simulink model "gauss_mf1_2"  (Simulink 7.2)
settings: Solver=ode45  StartTime=0.0  StopTime=10.0  RelTol=1e-3
values from neighbouring files (symbols this model uses):
  fi_1_mu = -0.7664    [fuzzy_controller_5_gauss_params.m]
  fi_1_sigma = 0.1502    [fuzzy_controller_5_gauss_params.m]
settings Model: Creator=Student  LastModifiedBy=Student  CovModelRefEnable=off
settings DataIOCC: LimitDataPoints=off  SaveFormat=StructureWithTime
settings OptimizationCC: ExpressionDepthLimit=128
settings DebuggingCC: UnderspecifiedInitializationDetection=Simplified  MergeDetectMultiDrivingBlocksExec=error  SolverPrmCheckMsg=none  FcnCallInpInsideContextMsg=Enable All  StateNameClashWarn=none  StrictBusMsg=ErrorLevel1
settings HardwareCC: ProdIntDivRoundTo=Zero  ProdEndianess=LittleEndian  ProdHWDeviceType=Specified
settings CodeAppCC: CustomSymbolStrType=$N$R$M_T
settings GRTTargetCC: TargetFunctionLibrary=C89/C90 (ANSI)

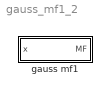
== system gauss_mf1_2 ==
  gauss mf1 : Subsystem  mask{sigma=fi_1_sigma, mu=fi_1_mu}
      mask prompts: sigma "Variance sigma:"; mu "Mean c:"

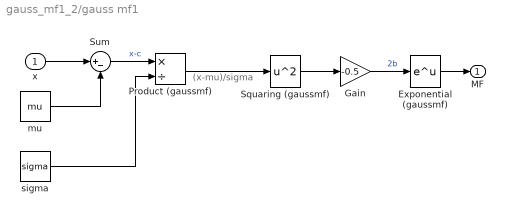
== system gauss_mf1_2/gauss mf1 ==
  note: (x-mu)/sigma
  x : Inport
  Exponential (gaussmf) : Math  SaturateOnIntegerOverflow=on
  Gain : Gain  Gain=-0.5  SaturateOnIntegerOverflow=on  OutDataTypeStr=Inherit: Same as input  ParamDataTypeStr=Inherit: Same as input
  Product (gaussmf) : Product  Inputs=*/  SaturateOnIntegerOverflow=on  InputSameDT=on  OutDataTypeStr=Inherit: Same as first input
  Squaring (gaussmf) : Math  Operator=square  SaturateOnIntegerOverflow=on
  Sum : Sum  Inputs=|+-  SaturateOnIntegerOverflow=on  InputSameDT=on  OutDataTypeStr=Inherit: Same as first input
  mu : Constant  Value=mu
  sigma : Constant  Value=sigma
  MF : Outport
  wires:
  Product (gaussmf)/1 -> Squaring (gaussmf)/1
  Gain/1 -> Exponential (gaussmf)/1  "2b"
  Squaring (gaussmf)/1 -> Gain/1
  Exponential (gaussmf)/1 -> MF/1
  sigma/1 -> Product (gaussmf)/2
  Sum/1 -> Product (gaussmf)/1  "x-c"
  mu/1 -> Sum/2
  x/1 -> Sum/1
